simulink model "Nonlinear_Observer_v2"  (R2021a)
settings: Solver=VariableStepAuto  StartTime=0.0  StopTime=20  RelTol=1e-3
settings Model: Creator=JianFongLee  LastModifiedBy=JianFongLee

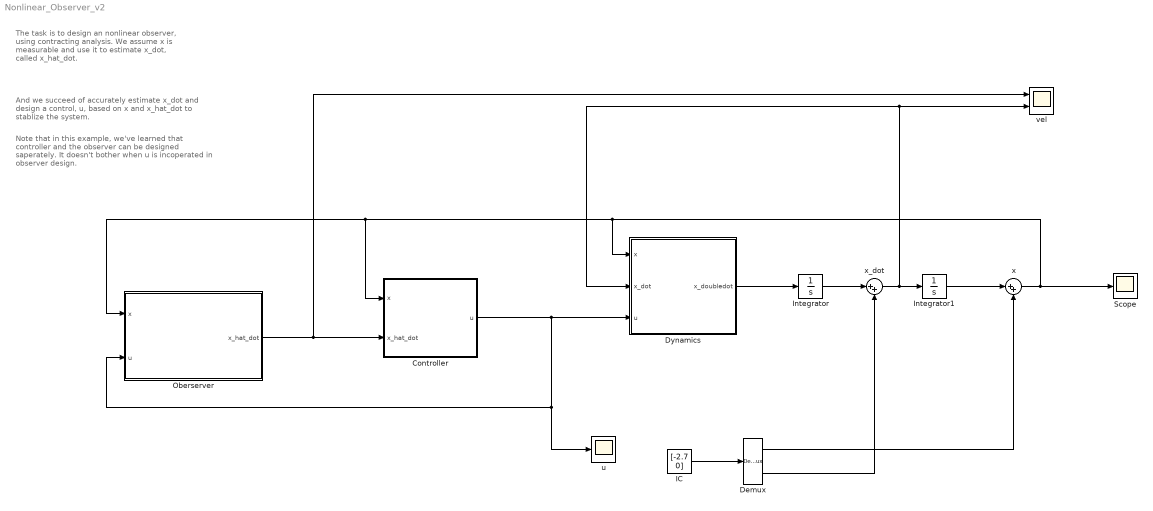
== system Nonlinear_Observer_v2 ==
  note: Note that in this example,
      | we've learned that controller and the observer
      | can be designed saperately.
      | It doesn't bother when u is incoperated in observer
      | design.
  note: And we succeed of accurately estimate x_dot
      | and design a control, u, based on x and x_hat_dot
      | to stablize the system.
  note: The task is to design an nonlinear observer,
      | using contracting analysis.
      | We assume x is measurable and use it to
      | estimate x_dot, called x_hat_dot.
  Controller : MATLAB Function  TreatAsAtomicUnit=on
  Demux : Demux  Outputs=2
      settings: DisplayOption=none
  Dynamics : MATLAB Function  TreatAsAtomicUnit=on
  IC : Constant  Value=[-2.7 0]
  Integrator : Integrator
  Integrator1 : Integrator
  Oberserver : Subsystem
  Scope : Scope
  u : Scope
  vel : Scope  NumInputPorts=2
  x : Sum  Inputs=|++
  x_dot : Sum  Inputs=|++
  wires:
  IC/1 -> Demux/1
  Dynamics/1(x_doubledot) -> Integrator/1
  Integrator/1 -> x_dot/1
  Demux/2 -> x_dot/2
  x_dot/1 -> vel/2, Dynamics/2(x_dot), Integrator1/1
  Integrator1/1 -> x/1
  Demux/1 -> x/2
  Controller/1(u) -> Oberserver/2(u), u/1, Dynamics/3(u)
  x/1 -> Scope/1, Controller/1(x), Oberserver/1(x), Dynamics/1(x)
  Oberserver/1(x_hat_dot) -> Controller/2(x_hat_dot), vel/1

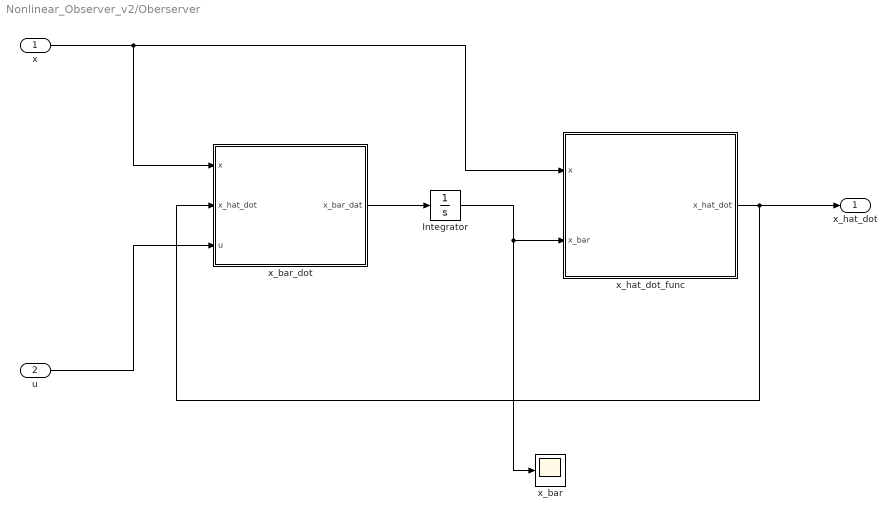
== system Nonlinear_Observer_v2/Oberserver ==
  x : Inport
  u : Inport  Port=2
  Integrator : Integrator
  x_bar : Scope
  x_bar_dot : MATLAB Function  TreatAsAtomicUnit=on
  x_hat_dot_func : MATLAB Function  TreatAsAtomicUnit=on
  x_hat_dot : Outport
  wires:
  x/1 -> x_bar_dot/1(x), x_hat_dot_func/1(x)
  u/1 -> x_bar_dot/3(u)
  x_bar_dot/1(x_bar_dat) -> Integrator/1
  Integrator/1 -> x_bar/1, x_hat_dot_func/2(x_bar)
  x_hat_dot_func/1(x_hat_dot) -> x_hat_dot/1, x_bar_dot/2(x_hat_dot)

== matlab function Nonlinear_Observer_v2/Dynamics ==
  data: x input; x_dot input; u input; x_doubledot output
function x_doubledot = fcn(x,x_dot,u)
%%% The dynamics of the system

x_doubledot = -x_dot*(x^2) - x_dot^3 + x*x + 7*x + u;
end

== matlab function Nonlinear_Observer_v2/Oberserver/x_bar_dot ==
  data: x input; x_hat_dot input; u input; x_bar_dat output
function x_bar_dat = fcn(x,x_hat_dot,u)

C = 0.001;  %%%should be greater than 0
   
x_bar_dat = -x_hat_dot*(x^2) - x_hat_dot^3 + x^2 ...
            + 7*x - C*x_hat_dot + u;
        
end

== matlab function Nonlinear_Observer_v2/Oberserver/x_hat_dot_func ==
  data: x input; x_bar input; x_hat_dot output
function x_hat_dot = fcn(x,x_bar)
%%%
C = 0.001; %%% Note the C should be consistent
x_hat_dot = C*x + x_bar;
end

== matlab function Nonlinear_Observer_v2/Controller ==
  data: x input; u output; x_hat_dot input
function u = fcn(x,x_hat_dot)
%%% Controller here
%%% Note that x_dot is not measureable,
%%% so we build a obersver for x_dot,called x_hat_dot
lemmda = 2;
R = 10;     %%%Restrain of u
s = x_hat_dot + lemmda*x;
k1 = 0.1;
u = -8*x-lemmda*x_hat_dot - x^2 + x_hat_dot^3 ...
    + x_hat_dot*(x^2) - k1*s;
% if(u>R)
%     u = R;
% elseif(u<-R)
%     u = -R;
% end
end
